simulink model "guzhangfangzhen"  (R2025a)
settings: Solver=VariableStepAuto  StartTime=0.0  StopTime=0.6  RelTol=1e-3
undefined symbols (not defined in the file or in its folder): D11, Delta
libraries: spsThreePhaseVIMeasurementLib x4, spsThreePhasePISectionLineLib x3, spsThreePhaseSeriesRLCLoadLib x3, spsThreePhaseSourceLib x1, spsGroundLib x1, spsSeriesRLCBranchLib x1, spsThreePhaseFaultLib x1, spsThreePhaseSeriesRLCBranchLib x1, spsThreePhaseTransformerTwoWindingsLib x1, spsZigzagPhaseShiftingTransformerLib x1, spspowerguiLib x1
settings Model: Creator=19092  LastModifiedBy=19092

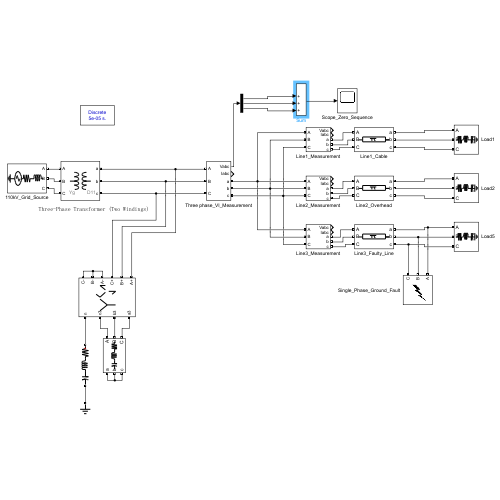
[thumbnail: Simulink's stored preview of the top-level diagram]
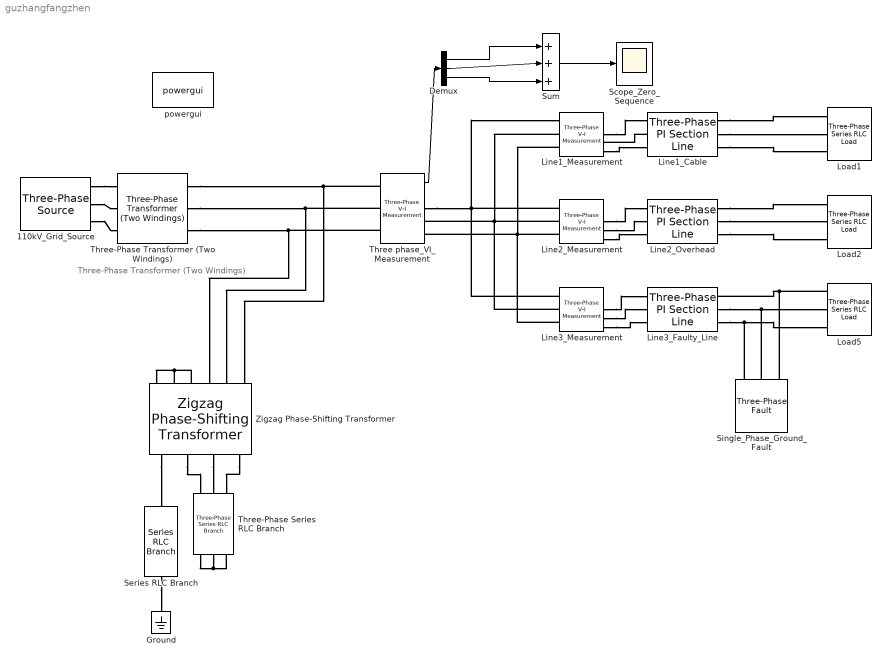
== system guzhangfangzhen ==
  note: Three-Phase Transformer (Two Windings)
  110kV_Grid_Source : spsThreePhaseSourceLib/Three-Phase Source  InternalConnection=Yg  VoltagePhases=off  Voltage=110e3  PhaseAngle=0  Voltage_phases=[25e3 25e3 25e3]/sqrt(3)  PhaseAngles_phases=[0 -120 +120]  Frequency=50  NonIdealSource=on  SpecifyImpedance=off  Resistance=0.8929  Inductance=16.58e-3  ShortCircuitLevel=100e6  BaseVoltage=110e3  XRratio=7  BusType=swing  Pref=10e3  Qref=0  Prefabc=[10e3, 10e3, 10e3]  Qrefabc=[0, 0, 0]  Qmin=-inf  Qmax=inf
  Demux : Demux  Outputs=3
  Ground : spsGroundLib/Ground  LConnTagsString=a
  Line1_Cable : spsThreePhasePISectionLineLib/Three-Phase PI Section Line  LConnTagsString=a|b|c  RConnTagsString=A|B|C  Length=100  Frequency=50  Resistances=[ 0.01273 0.3864]  Inductances="[ 0.9337e-3  4.1264e-3]"  Capacitances=[12.74e-9 7.751e-9]
  Line1_Measurement : spsThreePhaseVIMeasurementLib/Three-Phase V-I Measurement  VoltageMeasurement=phase-to-ground  SetLabelV=off  LabelV=Vabc  Vpu=off  VpuLL=off  CurrentMeasurement=yes  SetLabelI=off  LabelI=Iabc  Ipu=off  Pbase=100e6  Vbase=500e3  OutputType=Complex  PhasorSimulation=off  PSBequivalent=0
  Line2_Measurement : spsThreePhaseVIMeasurementLib/Three-Phase V-I Measurement  VoltageMeasurement=phase-to-ground  SetLabelV=off  LabelV=Vabc  Vpu=off  VpuLL=off  CurrentMeasurement=yes  SetLabelI=off  LabelI=Iabc  Ipu=off  Pbase=100e6  Vbase=500e3  OutputType=Complex  PhasorSimulation=off  PSBequivalent=0
  Line2_Overhead : spsThreePhasePISectionLineLib/Three-Phase PI Section Line  LConnTagsString=a|b|c  RConnTagsString=A|B|C  Length=100  Frequency=50  Resistances=[ 0.01273 0.3864]  Inductances="[ 0.9337e-3  4.1264e-3]"  Capacitances=[12.74e-9 7.751e-9]
  Line3_Faulty_Line : spsThreePhasePISectionLineLib/Three-Phase PI Section Line  LConnTagsString=a|b|c  RConnTagsString=A|B|C  Length=100  Frequency=50  Resistances=[ 0.01273 0.3864]  Inductances="[ 0.9337e-3  4.1264e-3]"  Capacitances=[12.74e-9 7.751e-9]
  Line3_Measurement : spsThreePhaseVIMeasurementLib/Three-Phase V-I Measurement  VoltageMeasurement=phase-to-ground  SetLabelV=off  LabelV=Vabc  Vpu=off  VpuLL=off  CurrentMeasurement=yes  SetLabelI=off  LabelI=Iabc  Ipu=off  Pbase=100e6  Vbase=500e3  OutputType=Complex  PhasorSimulation=off  PSBequivalent=0
  Load1 : spsThreePhaseSeriesRLCLoadLib/Three-Phase Series RLC Load  LConnTagsString=A|B|C  Configuration=Y (grounded)  NominalVoltage=1000  Vabc=[1e3 1e3 1e3]  Vabcp=[1e3 1e3 1e3]  NominalFrequency=50  UnbalancedPower=off  ActivePower=10e3  InductivePower=100  CapacitivePower=100  Pabc=[10e3 9e3 11e3]  QLabc=[100 90 110]  QCabc=[100 90 110]  Pabcp=[10e3 9e3 11e3]  QLabcp=[100 90 110]  QCabcp=[100 90 110]  Measurements=None  LoadType=constant Z
  Load2 : spsThreePhaseSeriesRLCLoadLib/Three-Phase Series RLC Load  LConnTagsString=A|B|C  Configuration=Y (grounded)  NominalVoltage=1000  Vabc=[1e3 1e3 1e3]  Vabcp=[1e3 1e3 1e3]  NominalFrequency=50  UnbalancedPower=off  ActivePower=10e3  InductivePower=100  CapacitivePower=100  Pabc=[10e3 9e3 11e3]  QLabc=[100 90 110]  QCabc=[100 90 110]  Pabcp=[10e3 9e3 11e3]  QLabcp=[100 90 110]  QCabcp=[100 90 110]  Measurements=None  LoadType=constant Z
  Load5 : spsThreePhaseSeriesRLCLoadLib/Three-Phase Series RLC Load  LConnTagsString=A|B|C  Configuration=Y (grounded)  NominalVoltage=1000  Vabc=[1e3 1e3 1e3]  Vabcp=[1e3 1e3 1e3]  NominalFrequency=50  UnbalancedPower=off  ActivePower=10e3  InductivePower=100  CapacitivePower=100  Pabc=[10e3 9e3 11e3]  QLabc=[100 90 110]  QCabc=[100 90 110]  Pabcp=[10e3 9e3 11e3]  QLabcp=[100 90 110]  QCabcp=[100 90 110]  Measurements=None  LoadType=constant Z
  Scope_Zero_Sequence : Scope
      settings: ActiveDisplayYMinimum=-11287.489482819756  ActiveDisplayYMaximum=9356.0828668048252
  Series RLC Branch : spsSeriesRLCBranchLib/Series RLC Branch  LConnTagsString=__new0  RConnTagsString=__new0  BranchType=RLC  Resistance=1  Inductance=1e-3  SetiL0=off  InitialCurrent=0  Capacitance=1e-6  Setx0=off  InitialVoltage=0  Measurements=None
  Single_Phase_Ground_Fault : spsThreePhaseFaultLib/Three-Phase Fault  InitialStates=0  FaultA=on  FaultB=off  FaultC=off  GroundFault=on  SwitchTimes="[0.2  0.3]"  External=off  SwitchStatus=NaN  FaultResistance=0.01  GroundResistance=0.01  SnubberResistance=1e6  SnubberCapacitance=inf  Measurements=None
  Sum : Sum  Inputs=|+++
  Three phase_VI_Measurement : spsThreePhaseVIMeasurementLib/Three-Phase V-I Measurement  VoltageMeasurement=phase-to-ground  SetLabelV=off  LabelV=Vabc  Vpu=off  VpuLL=off  CurrentMeasurement=yes  SetLabelI=off  LabelI=Iabc  Ipu=off  Pbase=100e6  Vbase=500e3  OutputType=Complex  PhasorSimulation=off  PSBequivalent=0
  Three-Phase Series RLC Branch : spsThreePhaseSeriesRLCBranchLib/Three-Phase Series RLC Branch  LConnTagsString=A|B|C  RConnTagsString=A|B|C  BranchType=RLC  Resistance=1  Inductance=1e-3  Capacitance=1e-6  Measurements=None
  Three-Phase Transformer (Two Windings) : spsThreePhaseTransformerTwoWindingsLib/Three-Phase Transformer (Two Windings)  Winding1Connection=Yg  Winding2Connection=Delta (D11)  CoreType=Three single-phase transformers  SetSaturation=off  Hysteresis=off  DataFile='hysteresis'  SetInitialFlux=off  Measurements=None  UNITS=pu  NominalPower=[ 20e6 , 50 ]  Winding1=[ 110e3 , 0.002 , 0.08 ]  Winding2=[ 10e3 , 0.002 , 0.08 ]  Rm=500  Lm=500  L0=0.5  Saturation=[ 0,0 ; 0.0024,1.2 ; 1.0,1.52 ]  InitialFluxes=[ 0.8 , -0.8 , 0.7 ]  BreakLoop=off  DiscreteSolver=Trapezoidal iterative  DataType=off  TransfoNumber=1
  Zigzag Phase-Shifting Transformer : spsZigzagPhaseShiftingTransformerLib/Zigzag Phase-Shifting Transformer  SecondaryConnection=Yn  SetSaturation=off  SetInitialFlux=off  Measurements=None  UNITS=pu  NominalPower=[ 100e6 50]  PrimaryVoltage=10e3  SecondaryVoltage="[ 30e3  +15]"  Winding1=[ 0.002 0.08 ]  Winding2="[ 0.002  0.08 ]"  Winding3=[ 0.002 0.08 ]  RmLm=[ 500 500 ]  Rm=500  Saturation=[ 0,0 ; 0.0024,1.2 ; 1.0,1.52 ]  InitialFluxes=[0,0,0]  BreakLoop=off  DiscreteSolver=Trapezoidal iterative  DataType=off
      settings: LibrarySourceBlock=|
      | sps_lib/Power Grid Elements/Zigzag
      | Phase-Shifting Transformer
  powergui : spspowerguiLib/powergui  Priority=1  SimulationMode=Discrete  SampleTime=50e-6  frequency=60  Iterations=50  frequencyindice=50  Pbase=100e6  ErrMax=1e-4  UnitsV=kV  UnitsW=MW  buscounter=0  FunctionMessages=off  echomessages=off  EnableUseOfTLC=off  CurrentSourceSwitches=off  DisableSnubberDevices=off  DisableRonSwitches=off  DisableVfSwitches=off  DisplayEquations=off  AutomaticDiscreteSolvers=off  SolverType=Tustin/Backward Euler (TBE)  Interpol=off  ExternalGateDelay=off  methode=off  Ts=100  x0status=blocks  SPID=on  SwTol=0  HookPort=off  NonlinearTolerance=1e-4  nMaxIteration=100  ContinueOnMaxIteration=off  RestoreLinks=warning  ResistiveCurrentMeasurement=off  Frange=[0:2:500]  Ylog=off  Xlog=on  ShowGrid=off  save=off  variable=ZData  structure=0  ZoomFFT=off  StartTime=0.0  cycles=1  DisplayStyle=1  fundamental=60  FreqAxis=off  MaxFrequency=1000  frequencyindicesteady=1  RmsSteady=1  display=off
  wires:
  Three phase_VI_Measurement/1 -> Demux/1
  Demux/1 -> Sum/1
  Demux/2 -> Sum/2
  Demux/3 -> Sum/3
  Sum/1 -> Scope_Zero_Sequence/1
  connections:
  110kV_Grid_Source/RConn1 -- Three-Phase Transformer (Two Windings)/LConn1
  110kV_Grid_Source/RConn2 -- Three-Phase Transformer (Two Windings)/LConn2
  110kV_Grid_Source/RConn3 -- Three-Phase Transformer (Two Windings)/LConn3
  Series RLC Branch/RConn1 -- Ground/LConn1
  Three-Phase Transformer (Two Windings)/RConn1 -- Three phase_VI_Measurement/LConn1 -- Zigzag Phase-Shifting Transformer/LConn1
  Three-Phase Transformer (Two Windings)/RConn2 -- Three phase_VI_Measurement/LConn2 -- Zigzag Phase-Shifting Transformer/LConn2
  Three-Phase Transformer (Two Windings)/RConn3 -- Three phase_VI_Measurement/LConn3 -- Zigzag Phase-Shifting Transformer/LConn3
  Zigzag Phase-Shifting Transformer/RConn4 -- Series RLC Branch/LConn1
  Zigzag Phase-Shifting Transformer/RConn3 -- Three-Phase Series RLC Branch/LConn1
  Zigzag Phase-Shifting Transformer/RConn2 -- Three-Phase Series RLC Branch/LConn2
  Zigzag Phase-Shifting Transformer/RConn1 -- Three-Phase Series RLC Branch/LConn3
  Three-Phase Series RLC Branch/RConn2 -- Three-Phase Series RLC Branch/RConn3 -- Three-Phase Series RLC Branch/RConn1
  Zigzag Phase-Shifting Transformer/LConn4 -- Zigzag Phase-Shifting Transformer/LConn6 -- Zigzag Phase-Shifting Transformer/LConn5
  Line1_Measurement/RConn1 -- Line1_Cable/LConn1
  Line1_Cable/LConn2 -- Line1_Measurement/RConn2
  Line1_Measurement/RConn3 -- Line1_Cable/LConn3
  Line1_Cable/RConn1 -- Load1/LConn1
  Line1_Cable/RConn2 -- Load1/LConn2
  Line1_Cable/RConn3 -- Load1/LConn3
  Line2_Measurement/RConn1 -- Line2_Overhead/LConn1
  Line2_Measurement/RConn2 -- Line2_Overhead/LConn2
  Line2_Measurement/RConn3 -- Line2_Overhead/LConn3
  Line2_Overhead/RConn1 -- Load2/LConn1
  Line2_Overhead/RConn2 -- Load2/LConn2
  Line2_Overhead/RConn3 -- Load2/LConn3
  Line3_Measurement/RConn1 -- Line3_Faulty_Line/LConn1
  Line3_Measurement/RConn2 -- Line3_Faulty_Line/LConn2
  Line3_Measurement/RConn3 -- Line3_Faulty_Line/LConn3
  Load5/LConn1 -- Single_Phase_Ground_Fault/LConn1 -- Line3_Faulty_Line/RConn1
  Line3_Faulty_Line/RConn2 -- Single_Phase_Ground_Fault/LConn2 -- Load5/LConn2
  Line3_Faulty_Line/RConn3 -- Single_Phase_Ground_Fault/LConn3 -- Load5/LConn3
  Three phase_VI_Measurement/RConn1 -- Line1_Measurement/LConn1 -- Line3_Measurement/LConn1 -- Line2_Measurement/LConn1
  Line1_Measurement/LConn2 -- Line2_Measurement/LConn2 -- Line3_Measurement/LConn2 -- Three phase_VI_Measurement/RConn2
  Line1_Measurement/LConn3 -- Three phase_VI_Measurement/RConn3 -- Line3_Measurement/LConn3 -- Line2_Measurement/LConn3
